simulink model "eVTOL_PX4_2023b"  (R2024b)
settings: Solver=ode4  StartTime=0  StopTime=inf  FixedStep=0.01  RelTol=1e-3
values from neighbouring files (symbols this model uses):
  aDl =     [initdata.mat]
  aDr =     [initdata.mat]
  aDyn =     [initdata.mat]
  Airport = init_airport('PHNL')    [initdata_HIL_eVTOL.m]
  aLat =     [initdata.mat]
  aLon =     [initdata.mat]
  D = Prop.D    [EOM_dt_MC.m]    (also in EOM_get_alf_dt_de_prop_evtol.m = CD * QS)
  dt0 = X(2)    [EOM_get_alf_dt_de_prop_evtol.m]    (also in initdata.mat = 0.258252593971; initdata_HIL_eVTOL.m = EOM_dt_MC)
  EAS0 = TAS0 / EAS2TAS    [initdata_HIL_eVTOL.m]
  FCS = init_FCS    [initdata_HIL_eVTOL.m]
  General = init_layoutdata    [EOM_dt_MC.m]    (also in build_optimized_CA.m; initdata.mat = ; initdata_HIL_eVTOL.m)
  h0 = Con(1)    [EOM_get_alf_dt_de_prop_evtol.m]    (also in initdata.mat = 450; initdata_HIL_eVTOL.m = 50)
  mass = Con(3)    [EOM_get_alf_dt_de_prop_evtol.m]    (also in initdata.mat = 2255.54; initdata_HIL_eVTOL.m = 7)
  Motor = init_motor_evtol    [EOM_dt_MC.m]    (also in initdata.mat = []; initdata_HIL_eVTOL.m)
  Prop = init_propeller_evtol_new    [EOM_dt_MC.m]    (also in initdata_HIL_eVTOL.m)
  R2D = 180/pi    (= 57.2957795131)    [EOM_get_alf_dt_de_prop_evtol.m]    (also in init_FCS.m; init_aerodata_evtol.m; init_airport.m; initdata.mat)
  SAMPLE_TIME = 0.01    [initdata_HIL_eVTOL.m]
  theta0 = -0.0510981441662    [initdata.mat]
undefined symbols (not defined in the file or in its folder): A1, aDa, aDe, aero, asbhl20env, B1, C1, de0, Earth, Environment, INIT_Data, InitData, Kd, Kp, magnitude, Newton, pProp, Raphson, Tc, WGS84
libraries: simulink_extras x63, vrlib x48, sharedtransform x28, simulink x22, slpidlib x20, sharedutil x20, matrix_library x18, aerolibwindfilters x12, aerolibobsolete x8, aerolibasang x8, aerolibatmos2 x6, aerolibfltsims x6
(part 16 of 17)

== system eVTOL_PX4_2023b/Subsystem2/airframe/force moment/aero F&M in body axis/Aerodynamic Coefficients/Body Rate Damping ==
  Incid : Inport
  pqrn : Inport  Port=2
  alphaDot_n : Inport  Port=3
  1-D Lookup Table : Lookup_n-D  NumberOfTableDimensions=1  BreakpointsForDimension1=aDyn.alpha  BreakpointsForDimension2=aDyn.flap  Table=aDyn.CYp  InternalRulePriority=Speed  RndMeth=Simplest
  1-D Lookup Table1 : Lookup_n-D  NumberOfTableDimensions=1  BreakpointsForDimension1=aDyn.alpha  BreakpointsForDimension2=aDyn.flap  Table=aDyn.Clp  InternalRulePriority=Speed  RndMeth=Simplest
  1-D Lookup Table2 : Lookup_n-D  NumberOfTableDimensions=1  BreakpointsForDimension1=aDyn.alpha  BreakpointsForDimension2=aDyn.flap  Table=aDyn.Cnp  InternalRulePriority=Speed  RndMeth=Simplest
  1-D Lookup Table3 : Lookup_n-D  NumberOfTableDimensions=1  BreakpointsForDimension1=aDyn.alpha  BreakpointsForDimension2=aDyn.flap  Table=aDyn.CYr  InternalRulePriority=Speed  RndMeth=Simplest
  1-D Lookup Table4 : Lookup_n-D  NumberOfTableDimensions=1  BreakpointsForDimension1=aDyn.alpha  BreakpointsForDimension2=aDyn.flap  Table=aDyn.Clr  InternalRulePriority=Speed  RndMeth=Simplest
  1-D Lookup Table5 : Lookup_n-D  NumberOfTableDimensions=1  BreakpointsForDimension1=aDyn.alpha  BreakpointsForDimension2=aDyn.flap  Table=aDyn.Cnr  InternalRulePriority=Speed  RndMeth=Simplest
  1-D Lookup Table6 : Lookup_n-D  NumberOfTableDimensions=1  BreakpointsForDimension1=aDyn.alpha  BreakpointsForDimension2=aDyn.flap  Table=aDyn.CLq  InternalRulePriority=Speed  RndMeth=Simplest
  1-D Lookup Table7 : Lookup_n-D  NumberOfTableDimensions=1  BreakpointsForDimension1=aDyn.alpha  BreakpointsForDimension2=aDyn.flap  Table=aDyn.Cmq  InternalRulePriority=Speed  RndMeth=Simplest
  1-D Lookup Table8 : Lookup_n-D  NumberOfTableDimensions=1  BreakpointsForDimension1=aDyn.alpha  BreakpointsForDimension2=aDyn.flap  Table=aDyn.CLAlphaDot  InternalRulePriority=Speed  RndMeth=Simplest
  1-D Lookup Table9 : Lookup_n-D  NumberOfTableDimensions=1  BreakpointsForDimension1=aDyn.alpha  BreakpointsForDimension2=aDyn.flap  Table=aDyn.CmAlphaDot  InternalRulePriority=Speed  RndMeth=Simplest
  Add : Sum  Inputs=++++
  Constant{,6..7,13} (4 alike) : Constant  Value=0
  Demux : Demux  Outputs=3
  Demux1 : Demux  Outputs=2
  Mux{1..4} (4 alike) : Mux  Inputs=6
  Product{4..7} (4 alike) : Product  InputSameDT=on  SaturateOnIntegerOverflow=on  OutDataTypeStr=Inherit: Same as first input
  Terminator : Terminator
  cl : Outport  InitialOutput=0  VectorParamsAs1DForOutWhenUnconnected=off
  wires:
  Add/1 -> cl/1
  1-D Lookup Table/1 -> Mux1/3  "CYp"
  1-D Lookup Table2/1 -> Mux1/6  "Cnp"
  Mux1/1 -> Product4/1
  1-D Lookup Table1/1 -> Mux1/4  "Clp"
  pqrn/1 -> Demux/1
  Demux/1 -> [p]
  Demux/2 -> [q]
  Demux/3 -> [r]
  Constant/1 -> Mux1/1, Mux1/2, Mux1/5
  1-D Lookup Table7/1 -> Mux2/5  "Cmq"
  1-D Lookup Table6/1 -> Mux2/1  "CLq"
  Mux2/1 -> Product5/1
  1-D Lookup Table3/1 -> Mux3/3  "CYr"
  Mux3/1 -> Product6/1
  1-D Lookup Table4/1 -> Mux3/4  "Clr"
  1-D Lookup Table5/1 -> Mux3/6  "Cnr"
  Constant7/1 -> Mux3/2, Mux3/5, Mux3/1
  Constant13/1 -> Mux4/6, Mux4/4, Mux4/3, Mux4/2
  1-D Lookup Table9/1 -> Mux4/5  "CmAlphaDot"
  1-D Lookup Table8/1 -> Mux4/1  "CLAlphaDot"
  Constant6/1 -> Mux2/4, Mux2/6, Mux2/3, Mux2/2
  [p] -> Product4/2
  [q] -> Product5/2
  [r] -> Product6/2
  Mux4/1 -> Product7/1
  alphaDot_n/1 -> Product7/2
  Product4/1 -> Add/1
  Product7/1 -> Add/4
  Demux1/2 -> Terminator/1  "beta"
  Demux1/1 -> [alpha]  "alpha"
  Incid/1 -> Demux1/1
  Product5/1 -> Add/3
  [alpha] -> 1-D Lookup Table3/1, 1-D Lookup Table4/1, 1-D Lookup Table9/1, 1-D Lookup Table8/1, 1-D Lookup Table7/1, 1-D Lookup Table6/1, 1-D Lookup Table5/1, 1-D Lookup Table2/1, 1-D Lookup Table1/1, 1-D Lookup Table/1
  Product6/1 -> Add/2

== system eVTOL_PX4_2023b/Subsystem2/airframe/force moment/aero F&M in body axis/Aerodynamic Coefficients/CLCDCY-CXCYCZ ==
  Incid : Inport
  Cl_LDY : Inport  Port=2
  Cl_xA : Fcn  Expr=-u[4]*cos(u[2])*cos(u[1])+u[3]*sin(u[1])
  Cl_yA : Fcn  Expr=-u[4]*sin(u[2])+u[5]
  Cl_zA : Fcn  Expr=-u[4]*cos(u[2])*sin(u[1])-u[3]*cos(u[1])
  Mux : Mux  Inputs=3
  Mux1 : Mux  Inputs=2
  Cl_XYZ : Outport  VectorParamsAs1DForOutWhenUnconnected=off
  wires:
  Mux/1 -> Cl_XYZ/1
  Cl_LDY/1 -> Mux1/2
  Incid/1 -> Mux1/1
  Cl_zA/1 -> Mux/3
  Cl_yA/1 -> Mux/2
  Cl_xA/1 -> Mux/1
  Mux1/1 -> Cl_zA/1, Cl_yA/1, Cl_xA/1

== system eVTOL_PX4_2023b/UAV/airframe/force moment/aero F&M in body axis/Aerodynamic Coefficients/Actuator Increments ==
  Actuators : Inport
  Aileron : Subsystem
  Bus Selector1 : BusSelector  OutputSignals=de,da,dr
  Elevator : Subsystem
  Ruder : Subsystem
  Sum : Sum  Inputs=+++
  da : Constant  Value=-1.25/57.3
  dr : Constant  Value=-6.3/57.3
  cl : Outport  InitialOutput=0  VectorParamsAs1DForOutWhenUnconnected=off
  wires:
  Actuators/1 -> Bus Selector1/1
  Bus Selector1/2 -> Aileron/1(da)  "<da>"
  Sum/1 -> cl/1
  Ruder/1(drCoeff) -> Sum/3
  Elevator/1(deCoeff) -> Sum/1
  Aileron/1(drCoeff) -> Sum/2
  Bus Selector1/1 -> Elevator/1(de)  "<de>"
  Bus Selector1/3 -> Ruder/1(dr)  "<dr>"

== system eVTOL_PX4_2023b/UAV/airframe/force moment/aero F&M in body axis/Aerodynamic Coefficients/Basic Coefficients ==
  Incid : Inport
  Constant : Constant  Value=aero.CL0
  Constant1 : Constant  Value=0
  Constant2 : Constant  Value=aero.CD0
  Constant3 : Constant  Value=aero.Cm0
  Constant4 : Constant  Value=0
  Demux : Demux  Outputs=2
  Gain : Gain  Gain=aero.CLAlpha
  Gain1 : Gain  Gain=aero.k
  Gain2 : Gain  Gain=aero.CmAlpha
  Gain3 : Gain  Gain=aero.CYBeta
  Gain4 : Gain  Gain=aero.ClBeta
  Gain5 : Gain  Gain=aero.CnBeta
  Mux1 : Mux  Inputs=6
  Mux2 : Mux  Inputs=6
  Product : Product
  Saturation : Saturate
  Saturation1 : Saturate  LowerLimit=-0.3
  Saturation2 : Saturate  UpperLimit=aero.CLMax  LowerLimit=-aero.CLMax
  Sum1 : Sum  Inputs=++|  InputSameDT=on  SaturateOnIntegerOverflow=on  OutDataTypeStr=Inherit: Same as first input
  Sum2 : Sum  Inputs=++|  InputSameDT=on  SaturateOnIntegerOverflow=on  OutDataTypeStr=Inherit: Same as first input
  Sum3 : Sum  Inputs=++|  InputSameDT=on  SaturateOnIntegerOverflow=on  OutDataTypeStr=Inherit: Same as first input
  Sum5 : Sum  Inputs=|++  InputSameDT=on  SaturateOnIntegerOverflow=on  OutDataTypeStr=Inherit: Same as first input
  cl : Outport  InitialOutput=0  VectorParamsAs1DForOutWhenUnconnected=off
  wires:
  Mux1/1 -> Sum5/1
  Demux/1 -> Saturation1/1  "alpha"
  Demux/2 -> Saturation/1  "beta"
  Sum2/1 -> Mux1/2
  Sum3/1 -> Mux1/5
  Sum1/1 -> Product/2, Product/1, Saturation2/1
  Constant1/1 -> Mux1/6, Mux1/4, Mux1/3
  Constant4/1 -> Mux2/5, Mux2/2, Mux2/1
  Gain3/1 -> Mux2/3
  Gain4/1 -> Mux2/4
  Gain5/1 -> Mux2/6
  Sum5/1 -> cl/1
  Mux2/1 -> Sum5/2
  Incid/1 -> Demux/1
  Saturation1/1 -> Gain2/1, Gain/1
  Saturation/1 -> Gain3/1, Gain5/1, Gain4/1
  Gain/1 -> Sum1/2
  Constant/1 -> Sum1/1
  Constant2/1 -> Sum2/1
  Product/1 -> Gain1/1
  Gain1/1 -> Sum2/2
  Constant3/1 -> Sum3/1
  Gain2/1 -> Sum3/2
  Saturation2/1 -> Mux1/1

== system eVTOL_PX4_2023b/UAV/airframe/force moment/aero F&M in body axis/Aerodynamic Coefficients/Body Rate Damping ==
  pqrn : Inport
  alphaDot_n : Inport  Port=2
  Demux : Demux  Outputs=3
  Product{,1..3} (4 alike) : Product  InputSameDT=on  SaturateOnIntegerOverflow=on  OutDataTypeStr=Inherit: Same as first input
  Sum1 : Sum  Inputs=++++  InputSameDT=on  SaturateOnIntegerOverflow=on  OutDataTypeStr=Inherit: Same as first input
  alphaDot : Subsystem
  p : Subsystem
  q : Subsystem
  r : Subsystem
  cl : Outport  InitialOutput=0  VectorParamsAs1DForOutWhenUnconnected=off
  wires:
  p/1(delCoeff) -> Product/1
  q/1(delCoeff) -> Product1/1
  Sum1/1 -> cl/1
  Product2/1 -> Sum1/3
  Product/1 -> Sum1/1
  r/1(delCoeff) -> Product2/1
  pqrn/1 -> Demux/1
  Demux/1 -> Product/2
  Demux/2 -> Product1/2
  Demux/3 -> Product2/2
  Product1/1 -> Sum1/2
  alphaDot/1(delCoeff) -> Product3/1
  alphaDot_n/1 -> Product3/2
  Product3/1 -> Sum1/4

== system eVTOL_PX4_2023b/UAV/airframe/force moment/aero F&M in body axis/Aerodynamic Coefficients/body axis forces ?????????? ==
  Incid : Inport
  Cl_LDY : Inport  Port=2
  Cl_xA : Fcn  Expr=-u[4]*cos(u[2])*cos(u[1])+u[3]*sin(u[1])
  Cl_yA : Fcn  Expr=-u[4]*sin(u[2])+u[5]
  Cl_zA : Fcn  Expr=-u[4]*cos(u[2])*sin(u[1])-u[3]*cos(u[1])
  Mux : Mux  Inputs=3
  Mux1 : Mux  Inputs=2
  Cl_XYZ : Outport  VectorParamsAs1DForOutWhenUnconnected=off
  wires:
  Mux/1 -> Cl_XYZ/1
  Cl_LDY/1 -> Mux1/2
  Incid/1 -> Mux1/1
  Cl_zA/1 -> Mux/3
  Cl_yA/1 -> Mux/2
  Cl_xA/1 -> Mux/1
  Mux1/1 -> Cl_zA/1, Cl_yA/1, Cl_xA/1

== system eVTOL_PX4_2023b/Subsystem1/Environment/Wind Models/Dryden Wind Turbulence Model (Continuous (+q -r))/Select angular rates/Interpolate rates/wind to body transformation ==
  DCM : Inport
  Wind direction : Inport  Port=2
  pg_l,qg_l,rg_l : Inport  Port=3
  Demux : Demux  Outputs=3
      settings: DisplayOption=none
  Product : Product  Multiplication=Matrix(*)  SaturateOnIntegerOverflow=on  OutDataTypeStr=Inherit: Same as first input
  Reshape : Reshape  OutputDimensionality=Customize  OutputDimensions=[3,1]
  Reshape1 : Reshape
  Vector Concatenate : Concatenate  NumInputs=3
  convert to earth coords : Subsystem
  pg,qg,rg : Outport  VectorParamsAs1DForOutWhenUnconnected=off
  wires:
  Reshape1/1 -> pg,qg,rg/1
  Reshape/1 -> Product/2
  DCM/1 -> Product/1
  Wind direction/1 -> convert to earth coords/1(Wind direction)
  convert to earth coords/1(pg) -> Vector Concatenate/1
  convert to earth coords/2(qg) -> Vector Concatenate/2
  Vector Concatenate/1 -> Reshape/1
  Demux/1 -> convert to earth coords/2(pg_l)
  Demux/2 -> convert to earth coords/3(qg_l)
  Demux/3 -> Vector Concatenate/3
  Product/1 -> Reshape1/1
  pg_l,qg_l,rg_l/1 -> Demux/1

== system eVTOL_PX4_2023b/Subsystem1/Environment/Wind Models/Dryden Wind Turbulence Model (Continuous (+q -r))/Select angular rates/Low altitude rates/wind to body transformation ==
  DCM : Inport
  Wind direction : Inport  Port=2
  pg_l,qg_l,rg_l : Inport  Port=3
  Demux : Demux  Outputs=3
      settings: DisplayOption=none
  Product : Product  Multiplication=Matrix(*)  SaturateOnIntegerOverflow=on  OutDataTypeStr=Inherit: Same as first input
  Reshape : Reshape  OutputDimensionality=Column vector (2-D)
  Reshape1 : Reshape
  Vector Concatenate : Concatenate  NumInputs=3
  convert to earth coords : Subsystem
  pg,qg,rg : Outport  VectorParamsAs1DForOutWhenUnconnected=off
  wires:
  pg_l,qg_l,rg_l/1 -> Demux/1
  Product/1 -> Reshape1/1
  Demux/3 -> Vector Concatenate/3
  Demux/2 -> convert to earth coords/3(qg_l)
  Demux/1 -> convert to earth coords/2(pg_l)
  Vector Concatenate/1 -> Reshape/1
  convert to earth coords/2(qg) -> Vector Concatenate/2
  convert to earth coords/1(pg) -> Vector Concatenate/1
  Wind direction/1 -> convert to earth coords/1(Wind direction)
  DCM/1 -> Product/1
  Reshape/1 -> Product/2
  Reshape1/1 -> pg,qg,rg/1

== system eVTOL_PX4_2023b/Subsystem1/Environment/Wind Models/Dryden Wind Turbulence Model (Continuous (+q -r))/Select velocities/Interpolate velocities/wind to body transformation ==
  DCM : Inport
  Wind direction : Inport  Port=2
  ug_l,vg_l,wg_l : Inport  Port=3
  Demux : Demux  Outputs=3
      settings: DisplayOption=none
  Product : Product  Multiplication=Matrix(*)  SaturateOnIntegerOverflow=on  OutDataTypeStr=Inherit: Same as first input
  Reshape : Reshape  OutputDimensionality=Customize  OutputDimensions=[3,1]
  Reshape1 : Reshape
  Vector Concatenate : Concatenate  NumInputs=3
  convert to earth coords : Subsystem
  ug,vg,wg : Outport  VectorParamsAs1DForOutWhenUnconnected=off
  wires:
  Reshape1/1 -> ug,vg,wg/1
  Reshape/1 -> Product/2
  ug_l,vg_l,wg_l/1 -> Demux/1
  Product/1 -> Reshape1/1
  Demux/3 -> Vector Concatenate/3
  Demux/2 -> convert to earth coords/3(vg_l)
  Demux/1 -> convert to earth coords/2(ug_l)
  Vector Concatenate/1 -> Reshape/1
  convert to earth coords/2(vg) -> Vector Concatenate/2
  convert to earth coords/1(ug) -> Vector Concatenate/1
  Wind direction/1 -> convert to earth coords/1(Wind direction)
  DCM/1 -> Product/1

== system eVTOL_PX4_2023b/Subsystem1/Environment/Wind Models/Dryden Wind Turbulence Model (Continuous (+q -r))/Select velocities/Low altitude velocities/wind to body transformation ==
  DCM : Inport
  Wind direction : Inport  Port=2
  ug_l,vg_l,wg_l : Inport  Port=3
  Demux : Demux  Outputs=3
      settings: DisplayOption=none
  Product : Product  Multiplication=Matrix(*)  SaturateOnIntegerOverflow=on  OutDataTypeStr=Inherit: Same as first input
  Reshape : Reshape  OutputDimensionality=Column vector (2-D)
  Reshape1 : Reshape
  Vector Concatenate : Concatenate  NumInputs=3
  convert to earth coords : Subsystem
  ug,vg,wg : Outport  VectorParamsAs1DForOutWhenUnconnected=off
  wires:
  DCM/1 -> Product/1
  Wind direction/1 -> convert to earth coords/1(Wind direction)
  convert to earth coords/1(ug) -> Vector Concatenate/1
  convert to earth coords/2(vg) -> Vector Concatenate/2
  Vector Concatenate/1 -> Reshape/1
  Demux/1 -> convert to earth coords/2(ug_l)
  Demux/2 -> convert to earth coords/3(vg_l)
  Demux/3 -> Vector Concatenate/3
  Product/1 -> Reshape1/1
  ug_l,vg_l,wg_l/1 -> Demux/1
  Reshape/1 -> Product/2
  Reshape1/1 -> ug,vg,wg/1

== system eVTOL_PX4_2023b/Subsystem1/Environment/Wind Models/Dryden Wind Turbulence Model (Continuous (+q -r))/Turbulence scale lengths/Medium//High altitude scale length/Length Conversion ==
  in : Inport  Unit=m
  Unit Conversion : UnitConversion
  out : Outport  VectorParamsAs1DForOutWhenUnconnected=off
  wires:
  in/1 -> Unit Conversion/1
  Unit Conversion/1 -> out/1

== system eVTOL_PX4_2023b/Subsystem1/Environment1/Wind Models/Dryden Wind Turbulence Model (Continuous (+q -r))/Select angular rates/Interpolate rates/wind to body transformation ==
  DCM : Inport
  Wind direction : Inport  Port=2
  pg_l,qg_l,rg_l : Inport  Port=3
  Demux : Demux  Outputs=3
      settings: DisplayOption=none
  Product : Product  Multiplication=Matrix(*)  SaturateOnIntegerOverflow=on  OutDataTypeStr=Inherit: Same as first input
  Reshape : Reshape  OutputDimensionality=Customize  OutputDimensions=[3,1]
  Reshape1 : Reshape
  Vector Concatenate : Concatenate  NumInputs=3
  convert to earth coords : Subsystem
  pg,qg,rg : Outport  VectorParamsAs1DForOutWhenUnconnected=off
  wires:
  Reshape1/1 -> pg,qg,rg/1
  Reshape/1 -> Product/2
  DCM/1 -> Product/1
  Wind direction/1 -> convert to earth coords/1(Wind direction)
  convert to earth coords/1(pg) -> Vector Concatenate/1
  convert to earth coords/2(qg) -> Vector Concatenate/2
  Vector Concatenate/1 -> Reshape/1
  Demux/1 -> convert to earth coords/2(pg_l)
  Demux/2 -> convert to earth coords/3(qg_l)
  Demux/3 -> Vector Concatenate/3
  Product/1 -> Reshape1/1
  pg_l,qg_l,rg_l/1 -> Demux/1

== system eVTOL_PX4_2023b/Subsystem1/Environment1/Wind Models/Dryden Wind Turbulence Model (Continuous (+q -r))/Select angular rates/Low altitude rates/wind to body transformation ==
  DCM : Inport
  Wind direction : Inport  Port=2
  pg_l,qg_l,rg_l : Inport  Port=3
  Demux : Demux  Outputs=3
      settings: DisplayOption=none
  Product : Product  Multiplication=Matrix(*)  SaturateOnIntegerOverflow=on  OutDataTypeStr=Inherit: Same as first input
  Reshape : Reshape  OutputDimensionality=Column vector (2-D)
  Reshape1 : Reshape
  Vector Concatenate : Concatenate  NumInputs=3
  convert to earth coords : Subsystem
  pg,qg,rg : Outport  VectorParamsAs1DForOutWhenUnconnected=off
  wires:
  pg_l,qg_l,rg_l/1 -> Demux/1
  Product/1 -> Reshape1/1
  Demux/3 -> Vector Concatenate/3
  Demux/2 -> convert to earth coords/3(qg_l)
  Demux/1 -> convert to earth coords/2(pg_l)
  Vector Concatenate/1 -> Reshape/1
  convert to earth coords/2(qg) -> Vector Concatenate/2
  convert to earth coords/1(pg) -> Vector Concatenate/1
  Wind direction/1 -> convert to earth coords/1(Wind direction)
  DCM/1 -> Product/1
  Reshape/1 -> Product/2
  Reshape1/1 -> pg,qg,rg/1

== system eVTOL_PX4_2023b/Subsystem1/Environment1/Wind Models/Dryden Wind Turbulence Model (Continuous (+q -r))/Select velocities/Interpolate velocities/wind to body transformation ==
  DCM : Inport
  Wind direction : Inport  Port=2
  ug_l,vg_l,wg_l : Inport  Port=3
  Demux : Demux  Outputs=3
      settings: DisplayOption=none
  Product : Product  Multiplication=Matrix(*)  SaturateOnIntegerOverflow=on  OutDataTypeStr=Inherit: Same as first input
  Reshape : Reshape  OutputDimensionality=Customize  OutputDimensions=[3,1]
  Reshape1 : Reshape
  Vector Concatenate : Concatenate  NumInputs=3
  convert to earth coords : Subsystem
  ug,vg,wg : Outport  VectorParamsAs1DForOutWhenUnconnected=off
  wires:
  Reshape1/1 -> ug,vg,wg/1
  Reshape/1 -> Product/2
  ug_l,vg_l,wg_l/1 -> Demux/1
  Product/1 -> Reshape1/1
  Demux/3 -> Vector Concatenate/3
  Demux/2 -> convert to earth coords/3(vg_l)
  Demux/1 -> convert to earth coords/2(ug_l)
  Vector Concatenate/1 -> Reshape/1
  convert to earth coords/2(vg) -> Vector Concatenate/2
  convert to earth coords/1(ug) -> Vector Concatenate/1
  Wind direction/1 -> convert to earth coords/1(Wind direction)
  DCM/1 -> Product/1

== system eVTOL_PX4_2023b/Subsystem1/Environment1/Wind Models/Dryden Wind Turbulence Model (Continuous (+q -r))/Select velocities/Low altitude velocities/wind to body transformation ==
  DCM : Inport
  Wind direction : Inport  Port=2
  ug_l,vg_l,wg_l : Inport  Port=3
  Demux : Demux  Outputs=3
      settings: DisplayOption=none
  Product : Product  Multiplication=Matrix(*)  SaturateOnIntegerOverflow=on  OutDataTypeStr=Inherit: Same as first input
  Reshape : Reshape  OutputDimensionality=Column vector (2-D)
  Reshape1 : Reshape
  Vector Concatenate : Concatenate  NumInputs=3
  convert to earth coords : Subsystem
  ug,vg,wg : Outport  VectorParamsAs1DForOutWhenUnconnected=off
  wires:
  DCM/1 -> Product/1
  Wind direction/1 -> convert to earth coords/1(Wind direction)
  convert to earth coords/1(ug) -> Vector Concatenate/1
  convert to earth coords/2(vg) -> Vector Concatenate/2
  Vector Concatenate/1 -> Reshape/1
  Demux/1 -> convert to earth coords/2(ug_l)
  Demux/2 -> convert to earth coords/3(vg_l)
  Demux/3 -> Vector Concatenate/3
  Product/1 -> Reshape1/1
  ug_l,vg_l,wg_l/1 -> Demux/1
  Reshape/1 -> Product/2
  Reshape1/1 -> ug,vg,wg/1

== system eVTOL_PX4_2023b/Subsystem1/Environment1/Wind Models/Dryden Wind Turbulence Model (Continuous (+q -r))/Turbulence scale lengths/Medium//High altitude scale length/Length Conversion ==
  in : Inport  Unit=m
  Unit Conversion : UnitConversion
  out : Outport  VectorParamsAs1DForOutWhenUnconnected=off
  wires:
  in/1 -> Unit Conversion/1
  Unit Conversion/1 -> out/1

== system eVTOL_PX4_2023b/Subsystem1/airframe/force moment/aero F&M in body axis/Aerodynamic Coefficients/Actuator Increments/Aileron ==
  alpha : Inport
  da : Inport  Port=2
  2-D Lookup Table3 : Lookup_n-D  NumberOfTableDimensions=1  BreakpointsForDimension1=aDa.alpha  BreakpointsForDimension2=aDe.alpha  BreakpointsForDimension3=aDe.flap  Table=aDa.CYDa  InternalRulePriority=Speed  RndMeth=Simplest
  2-D Lookup Table4 : Lookup_n-D  NumberOfTableDimensions=1  BreakpointsForDimension1=aDa.alpha  BreakpointsForDimension2=aDe.alpha  BreakpointsForDimension3=aDe.flap  Table=aDa.ClDa  InternalRulePriority=Speed  RndMeth=Simplest
  2-D Lookup Table5 : Lookup_n-D  NumberOfTableDimensions=1  BreakpointsForDimension1=aDa.alpha  BreakpointsForDimension2=aDe.alpha  BreakpointsForDimension3=aDe.flap  Table=aDa.CnDa  InternalRulePriority=Speed  RndMeth=Simplest
  Constant : Constant  Value=0
  Divide2 : Product  Inputs=**
  Divide3 : Product  Inputs=**
  Divide5 : Product  Inputs=**
  Mux1 : Mux  Inputs=6
  Saturation : Saturate  UpperLimit=12/57.3  LowerLimit=-4/57.3
  da_Coeff : Outport  VectorParamsAs1DForOutWhenUnconnected=off
  wires:
  alpha/1 -> Saturation/1
  Mux1/1 -> da_Coeff/1
  da/1 -> Divide5/1, Divide3/1, Divide2/1
  Divide2/1 -> Mux1/3
  Divide3/1 -> Mux1/4
  2-D Lookup Table3/1 -> Divide2/2
  Divide5/1 -> Mux1/6
  2-D Lookup Table5/1 -> Divide5/2
  2-D Lookup Table4/1 -> Divide3/2
  Constant/1 -> Mux1/5, Mux1/2, Mux1/1
  Saturation/1 -> 2-D Lookup Table5/1, 2-D Lookup Table4/1, 2-D Lookup Table3/1

== system eVTOL_PX4_2023b/Subsystem1/airframe/force moment/aero F&M in body axis/Aerodynamic Coefficients/Actuator Increments/V_left ==
  alpha : Inport
  dl : Inport  Port=2
  2-D Lookup Table : Lookup_n-D  NumberOfTableDimensions=1  BreakpointsForDimension1=aDl.alpha  BreakpointsForDimension2=aDl.alpha  BreakpointsForDimension3=aDe.flap  Table=aDl.CLDl  InternalRulePriority=Speed  RndMeth=Simplest
  2-D Lookup Table1 : Lookup_n-D  NumberOfTableDimensions=1  BreakpointsForDimension1=aDl.alpha  BreakpointsForDimension2=aDe.alpha  BreakpointsForDimension3=aDe.flap  Table=aDl.CmDl  InternalRulePriority=Speed  RndMeth=Simplest
  2-D Lookup Table2 : Lookup_n-D  NumberOfTableDimensions=1  BreakpointsForDimension1=aDl.alpha  BreakpointsForDimension2=aDe.alpha  BreakpointsForDimension3=aDe.flap  Table=aDl.CDDl  InternalRulePriority=Speed  RndMeth=Simplest
  2-D Lookup Table3 : Lookup_n-D  NumberOfTableDimensions=1  BreakpointsForDimension1=aDl.alpha  BreakpointsForDimension2=aDe.alpha  BreakpointsForDimension3=aDe.flap  Table=aDl.CYDl  InternalRulePriority=Speed  RndMeth=Simplest
  2-D Lookup Table4 : Lookup_n-D  NumberOfTableDimensions=1  BreakpointsForDimension1=aDl.alpha  BreakpointsForDimension2=aDe.alpha  BreakpointsForDimension3=aDe.flap  Table=aDl.ClDl  InternalRulePriority=Speed  RndMeth=Simplest
  2-D Lookup Table5 : Lookup_n-D  NumberOfTableDimensions=1  BreakpointsForDimension1=aDl.alpha  BreakpointsForDimension2=aDe.alpha  BreakpointsForDimension3=aDe.flap  Table=aDl.CnDl  InternalRulePriority=Speed  RndMeth=Simplest
  Divide{,1..5} (6 alike) : Product  Inputs=**
  Mux1 : Mux  Inputs=6
  Saturation : Saturate  UpperLimit=12/57.3  LowerLimit=-4/57.3
  dl_Coeff : Outport  VectorParamsAs1DForOutWhenUnconnected=off
  wires:
  2-D Lookup Table/1 -> Divide/2
  2-D Lookup Table2/1 -> Divide1/2
  2-D Lookup Table1/1 -> Divide4/2
  Mux1/1 -> dl_Coeff/1
  Divide4/1 -> Mux1/5
  Divide/1 -> Mux1/1
  Divide1/1 -> Mux1/2
  Divide2/1 -> Mux1/3
  2-D Lookup Table3/1 -> Divide2/2
  Divide3/1 -> Mux1/4
  2-D Lookup Table4/1 -> Divide3/2
  dl/1 -> Divide5/1, Divide4/1, Divide3/1, Divide2/1, Divide1/1, Divide/1
  alpha/1 -> Saturation/1
  2-D Lookup Table5/1 -> Divide5/2
  Divide5/1 -> Mux1/6
  Saturation/1 -> 2-D Lookup Table5/1, 2-D Lookup Table1/1, 2-D Lookup Table4/1, 2-D Lookup Table3/1, 2-D Lookup Table2/1, 2-D Lookup Table/1

== system eVTOL_PX4_2023b/Subsystem1/airframe/force moment/aero F&M in body axis/Aerodynamic Coefficients/Actuator Increments/V_right ==
  alpha : Inport
  dr : Inport  Port=2
  2-D Lookup Table : Lookup_n-D  NumberOfTableDimensions=1  BreakpointsForDimension1=aDr.alpha  BreakpointsForDimension2=aDl.alpha  BreakpointsForDimension3=aDe.flap  Table=aDr.CLDr  InternalRulePriority=Speed  RndMeth=Simplest
  2-D Lookup Table1 : Lookup_n-D  NumberOfTableDimensions=1  BreakpointsForDimension1=aDr.alpha  BreakpointsForDimension2=aDe.alpha  BreakpointsForDimension3=aDe.flap  Table=aDr.CmDr  InternalRulePriority=Speed  RndMeth=Simplest
  2-D Lookup Table2 : Lookup_n-D  NumberOfTableDimensions=1  BreakpointsForDimension1=aDr.alpha  BreakpointsForDimension2=aDe.alpha  BreakpointsForDimension3=aDe.flap  Table=aDr.CDDr  InternalRulePriority=Speed  RndMeth=Simplest
  2-D Lookup Table3 : Lookup_n-D  NumberOfTableDimensions=1  BreakpointsForDimension1=aDr.alpha  BreakpointsForDimension2=aDe.alpha  BreakpointsForDimension3=aDe.flap  Table=aDr.CYDr  InternalRulePriority=Speed  RndMeth=Simplest
  2-D Lookup Table4 : Lookup_n-D  NumberOfTableDimensions=1  BreakpointsForDimension1=aDr.alpha  BreakpointsForDimension2=aDe.alpha  BreakpointsForDimension3=aDe.flap  Table=aDr.ClDr  InternalRulePriority=Speed  RndMeth=Simplest
  2-D Lookup Table5 : Lookup_n-D  NumberOfTableDimensions=1  BreakpointsForDimension1=aDr.alpha  BreakpointsForDimension2=aDe.alpha  BreakpointsForDimension3=aDe.flap  Table=aDr.CnDr  InternalRulePriority=Speed  RndMeth=Simplest
  Divide{,1..5} (6 alike) : Product  Inputs=**
  Mux1 : Mux  Inputs=6
  Saturation : Saturate  UpperLimit=12/57.3  LowerLimit=-4/57.3
  dr_Coeff : Outport  VectorParamsAs1DForOutWhenUnconnected=off
  wires:
  dr/1 -> Divide5/1, Divide4/1, Divide3/1, Divide2/1, Divide1/1, Divide/1
  alpha/1 -> Saturation/1
  Divide/1 -> Mux1/1
  2-D Lookup Table5/1 -> Divide5/2
  Divide5/1 -> Mux1/6
  2-D Lookup Table1/1 -> Divide4/2
  Divide4/1 -> Mux1/5
  Divide2/1 -> Mux1/3
  2-D Lookup Table4/1 -> Divide3/2
  2-D Lookup Table/1 -> Divide/2
  2-D Lookup Table3/1 -> Divide2/2
  Mux1/1 -> dr_Coeff/1
  Divide3/1 -> Mux1/4
  2-D Lookup Table2/1 -> Divide1/2
  Divide1/1 -> Mux1/2
  Saturation/1 -> 2-D Lookup Table5/1, 2-D Lookup Table1/1, 2-D Lookup Table4/1, 2-D Lookup Table3/1, 2-D Lookup Table2/1, 2-D Lookup Table/1

== system eVTOL_PX4_2023b/Subsystem1/airframe1/force moment/aero F&M in body axis/Aerodynamic Coefficients/Actuator Increments/Aileron ==
  alpha : Inport
  da : Inport  Port=2
  2-D Lookup Table3 : Lookup_n-D  NumberOfTableDimensions=1  BreakpointsForDimension1=aDa.alpha  BreakpointsForDimension2=aDe.alpha  BreakpointsForDimension3=aDe.flap  Table=aDa.CYDa  InternalRulePriority=Speed  RndMeth=Simplest
  2-D Lookup Table4 : Lookup_n-D  NumberOfTableDimensions=1  BreakpointsForDimension1=aDa.alpha  BreakpointsForDimension2=aDe.alpha  BreakpointsForDimension3=aDe.flap  Table=aDa.ClDa  InternalRulePriority=Speed  RndMeth=Simplest
  2-D Lookup Table5 : Lookup_n-D  NumberOfTableDimensions=1  BreakpointsForDimension1=aDa.alpha  BreakpointsForDimension2=aDe.alpha  BreakpointsForDimension3=aDe.flap  Table=aDa.CnDa  InternalRulePriority=Speed  RndMeth=Simplest
  Constant : Constant  Value=0
  Divide2 : Product  Inputs=**
  Divide3 : Product  Inputs=**
  Divide5 : Product  Inputs=**
  Mux1 : Mux  Inputs=6
  da_Coeff : Outport  VectorParamsAs1DForOutWhenUnconnected=off
  wires:
  alpha/1 -> 2-D Lookup Table5/1, 2-D Lookup Table4/1, 2-D Lookup Table3/1
  Mux1/1 -> da_Coeff/1
  da/1 -> Divide5/1, Divide3/1, Divide2/1
  Divide2/1 -> Mux1/3
  Divide3/1 -> Mux1/4
  2-D Lookup Table3/1 -> Divide2/2
  Divide5/1 -> Mux1/6
  2-D Lookup Table5/1 -> Divide5/2
  2-D Lookup Table4/1 -> Divide3/2
  Constant/1 -> Mux1/5, Mux1/2, Mux1/1

== system eVTOL_PX4_2023b/Subsystem1/airframe1/force moment/aero F&M in body axis/Aerodynamic Coefficients/Actuator Increments/V_left ==
  alpha : Inport
  dl : Inport  Port=2
  2-D Lookup Table : Lookup_n-D  NumberOfTableDimensions=1  BreakpointsForDimension1=aDl.alpha  BreakpointsForDimension2=aDl.alpha  BreakpointsForDimension3=aDe.flap  Table=aDl.CLDl  InternalRulePriority=Speed  RndMeth=Simplest
  2-D Lookup Table1 : Lookup_n-D  NumberOfTableDimensions=1  BreakpointsForDimension1=aDl.alpha  BreakpointsForDimension2=aDe.alpha  BreakpointsForDimension3=aDe.flap  Table=aDl.CmDl  InternalRulePriority=Speed  RndMeth=Simplest
  2-D Lookup Table2 : Lookup_n-D  NumberOfTableDimensions=1  BreakpointsForDimension1=aDl.alpha  BreakpointsForDimension2=aDe.alpha  BreakpointsForDimension3=aDe.flap  Table=aDl.CDDl  InternalRulePriority=Speed  RndMeth=Simplest
  2-D Lookup Table3 : Lookup_n-D  NumberOfTableDimensions=1  BreakpointsForDimension1=aDl.alpha  BreakpointsForDimension2=aDe.alpha  BreakpointsForDimension3=aDe.flap  Table=aDl.CYDl  InternalRulePriority=Speed  RndMeth=Simplest
  2-D Lookup Table4 : Lookup_n-D  NumberOfTableDimensions=1  BreakpointsForDimension1=aDl.alpha  BreakpointsForDimension2=aDe.alpha  BreakpointsForDimension3=aDe.flap  Table=aDl.ClDl  InternalRulePriority=Speed  RndMeth=Simplest
  2-D Lookup Table5 : Lookup_n-D  NumberOfTableDimensions=1  BreakpointsForDimension1=aDl.alpha  BreakpointsForDimension2=aDe.alpha  BreakpointsForDimension3=aDe.flap  Table=aDl.CnDl  InternalRulePriority=Speed  RndMeth=Simplest
  Divide{,1..5} (6 alike) : Product  Inputs=**
  Mux1 : Mux  Inputs=6
  dl_Coeff : Outport  VectorParamsAs1DForOutWhenUnconnected=off
  wires:
  2-D Lookup Table/1 -> Divide/2
  2-D Lookup Table2/1 -> Divide1/2
  2-D Lookup Table1/1 -> Divide4/2
  Mux1/1 -> dl_Coeff/1
  Divide4/1 -> Mux1/5
  Divide/1 -> Mux1/1
  Divide1/1 -> Mux1/2
  Divide2/1 -> Mux1/3
  2-D Lookup Table3/1 -> Divide2/2
  Divide3/1 -> Mux1/4
  2-D Lookup Table4/1 -> Divide3/2
  dl/1 -> Divide5/1, Divide4/1, Divide3/1, Divide2/1, Divide1/1, Divide/1
  alpha/1 -> 2-D Lookup Table5/1, 2-D Lookup Table1/1, 2-D Lookup Table4/1, 2-D Lookup Table3/1, 2-D Lookup Table2/1, 2-D Lookup Table/1
  2-D Lookup Table5/1 -> Divide5/2
  Divide5/1 -> Mux1/6

== system eVTOL_PX4_2023b/Subsystem1/airframe1/force moment/aero F&M in body axis/Aerodynamic Coefficients/Actuator Increments/V_right ==
  alpha : Inport
  dr : Inport  Port=2
  2-D Lookup Table : Lookup_n-D  NumberOfTableDimensions=1  BreakpointsForDimension1=aDr.alpha  BreakpointsForDimension2=aDl.alpha  BreakpointsForDimension3=aDe.flap  Table=aDr.CLDr  InternalRulePriority=Speed  RndMeth=Simplest
  2-D Lookup Table1 : Lookup_n-D  NumberOfTableDimensions=1  BreakpointsForDimension1=aDr.alpha  BreakpointsForDimension2=aDe.alpha  BreakpointsForDimension3=aDe.flap  Table=aDr.CmDr  InternalRulePriority=Speed  RndMeth=Simplest
  2-D Lookup Table2 : Lookup_n-D  NumberOfTableDimensions=1  BreakpointsForDimension1=aDr.alpha  BreakpointsForDimension2=aDe.alpha  BreakpointsForDimension3=aDe.flap  Table=aDr.CDDr  InternalRulePriority=Speed  RndMeth=Simplest
  2-D Lookup Table3 : Lookup_n-D  NumberOfTableDimensions=1  BreakpointsForDimension1=aDr.alpha  BreakpointsForDimension2=aDe.alpha  BreakpointsForDimension3=aDe.flap  Table=aDr.CYDr  InternalRulePriority=Speed  RndMeth=Simplest
  2-D Lookup Table4 : Lookup_n-D  NumberOfTableDimensions=1  BreakpointsForDimension1=aDr.alpha  BreakpointsForDimension2=aDe.alpha  BreakpointsForDimension3=aDe.flap  Table=aDr.ClDr  InternalRulePriority=Speed  RndMeth=Simplest
  2-D Lookup Table5 : Lookup_n-D  NumberOfTableDimensions=1  BreakpointsForDimension1=aDr.alpha  BreakpointsForDimension2=aDe.alpha  BreakpointsForDimension3=aDe.flap  Table=aDr.CnDr  InternalRulePriority=Speed  RndMeth=Simplest
  Divide{,1..5} (6 alike) : Product  Inputs=**
  Mux1 : Mux  Inputs=6
  dr_Coeff : Outport  VectorParamsAs1DForOutWhenUnconnected=off
  wires:
  dr/1 -> Divide5/1, Divide4/1, Divide3/1, Divide2/1, Divide1/1, Divide/1
  alpha/1 -> 2-D Lookup Table5/1, 2-D Lookup Table1/1, 2-D Lookup Table4/1, 2-D Lookup Table3/1, 2-D Lookup Table2/1, 2-D Lookup Table/1
  Divide/1 -> Mux1/1
  2-D Lookup Table5/1 -> Divide5/2
  Divide5/1 -> Mux1/6
  2-D Lookup Table1/1 -> Divide4/2
  Divide4/1 -> Mux1/5
  Divide2/1 -> Mux1/3
  2-D Lookup Table4/1 -> Divide3/2
  2-D Lookup Table/1 -> Divide/2
  2-D Lookup Table3/1 -> Divide2/2
  Mux1/1 -> dr_Coeff/1
  Divide3/1 -> Mux1/4
  2-D Lookup Table2/1 -> Divide1/2
  Divide1/1 -> Mux1/2

== system eVTOL_PX4_2023b/Subsystem2/Environment/Wind Models/Dryden Wind Turbulence Model (Continuous (+q -r))/Select angular rates/Interpolate rates/wind to body transformation ==
  DCM : Inport
  Wind direction : Inport  Port=2
  pg_l,qg_l,rg_l : Inport  Port=3
  Demux : Demux  Outputs=3
      settings: DisplayOption=none
  Product : Product  Multiplication=Matrix(*)  SaturateOnIntegerOverflow=on  OutDataTypeStr=Inherit: Same as first input
  Reshape : Reshape  OutputDimensionality=Customize  OutputDimensions=[3,1]
  Reshape1 : Reshape
  Vector Concatenate : Concatenate  NumInputs=3
  convert to earth coords : Subsystem
  pg,qg,rg : Outport  VectorParamsAs1DForOutWhenUnconnected=off
  wires:
  Reshape1/1 -> pg,qg,rg/1
  Reshape/1 -> Product/2
  DCM/1 -> Product/1
  Wind direction/1 -> convert to earth coords/1(Wind direction)
  convert to earth coords/1(pg) -> Vector Concatenate/1
  convert to earth coords/2(qg) -> Vector Concatenate/2
  Vector Concatenate/1 -> Reshape/1
  Demux/1 -> convert to earth coords/2(pg_l)
  Demux/2 -> convert to earth coords/3(qg_l)
  Demux/3 -> Vector Concatenate/3
  Product/1 -> Reshape1/1
  pg_l,qg_l,rg_l/1 -> Demux/1

== system eVTOL_PX4_2023b/Subsystem2/Environment/Wind Models/Dryden Wind Turbulence Model (Continuous (+q -r))/Select angular rates/Low altitude rates/wind to body transformation ==
  DCM : Inport
  Wind direction : Inport  Port=2
  pg_l,qg_l,rg_l : Inport  Port=3
  Demux : Demux  Outputs=3
      settings: DisplayOption=none
  Product : Product  Multiplication=Matrix(*)  SaturateOnIntegerOverflow=on  OutDataTypeStr=Inherit: Same as first input
  Reshape : Reshape  OutputDimensionality=Column vector (2-D)
  Reshape1 : Reshape
  Vector Concatenate : Concatenate  NumInputs=3
  convert to earth coords : Subsystem
  pg,qg,rg : Outport  VectorParamsAs1DForOutWhenUnconnected=off
  wires:
  pg_l,qg_l,rg_l/1 -> Demux/1
  Product/1 -> Reshape1/1
  Demux/3 -> Vector Concatenate/3
  Demux/2 -> convert to earth coords/3(qg_l)
  Demux/1 -> convert to earth coords/2(pg_l)
  Vector Concatenate/1 -> Reshape/1
  convert to earth coords/2(qg) -> Vector Concatenate/2
  convert to earth coords/1(pg) -> Vector Concatenate/1
  Wind direction/1 -> convert to earth coords/1(Wind direction)
  DCM/1 -> Product/1
  Reshape/1 -> Product/2
  Reshape1/1 -> pg,qg,rg/1

== system eVTOL_PX4_2023b/Subsystem2/Environment/Wind Models/Dryden Wind Turbulence Model (Continuous (+q -r))/Select velocities/Interpolate velocities/wind to body transformation ==
  DCM : Inport
  Wind direction : Inport  Port=2
  ug_l,vg_l,wg_l : Inport  Port=3
  Demux : Demux  Outputs=3
      settings: DisplayOption=none
  Product : Product  Multiplication=Matrix(*)  SaturateOnIntegerOverflow=on  OutDataTypeStr=Inherit: Same as first input
  Reshape : Reshape  OutputDimensionality=Customize  OutputDimensions=[3,1]
  Reshape1 : Reshape
  Vector Concatenate : Concatenate  NumInputs=3
  convert to earth coords : Subsystem
  ug,vg,wg : Outport  VectorParamsAs1DForOutWhenUnconnected=off
  wires:
  Reshape1/1 -> ug,vg,wg/1
  Reshape/1 -> Product/2
  ug_l,vg_l,wg_l/1 -> Demux/1
  Product/1 -> Reshape1/1
  Demux/3 -> Vector Concatenate/3
  Demux/2 -> convert to earth coords/3(vg_l)
  Demux/1 -> convert to earth coords/2(ug_l)
  Vector Concatenate/1 -> Reshape/1
  convert to earth coords/2(vg) -> Vector Concatenate/2
  convert to earth coords/1(ug) -> Vector Concatenate/1
  Wind direction/1 -> convert to earth coords/1(Wind direction)
  DCM/1 -> Product/1

== system eVTOL_PX4_2023b/Subsystem2/Environment/Wind Models/Dryden Wind Turbulence Model (Continuous (+q -r))/Select velocities/Low altitude velocities/wind to body transformation ==
  DCM : Inport
  Wind direction : Inport  Port=2
  ug_l,vg_l,wg_l : Inport  Port=3
  Demux : Demux  Outputs=3
      settings: DisplayOption=none
  Product : Product  Multiplication=Matrix(*)  SaturateOnIntegerOverflow=on  OutDataTypeStr=Inherit: Same as first input
  Reshape : Reshape  OutputDimensionality=Column vector (2-D)
  Reshape1 : Reshape
  Vector Concatenate : Concatenate  NumInputs=3
  convert to earth coords : Subsystem
  ug,vg,wg : Outport  VectorParamsAs1DForOutWhenUnconnected=off
  wires:
  DCM/1 -> Product/1
  Wind direction/1 -> convert to earth coords/1(Wind direction)
  convert to earth coords/1(ug) -> Vector Concatenate/1
  convert to earth coords/2(vg) -> Vector Concatenate/2
  Vector Concatenate/1 -> Reshape/1
  Demux/1 -> convert to earth coords/2(ug_l)
  Demux/2 -> convert to earth coords/3(vg_l)
  Demux/3 -> Vector Concatenate/3
  Product/1 -> Reshape1/1
  ug_l,vg_l,wg_l/1 -> Demux/1
  Reshape/1 -> Product/2
  Reshape1/1 -> ug,vg,wg/1

== system eVTOL_PX4_2023b/Subsystem2/Environment/Wind Models/Dryden Wind Turbulence Model (Continuous (+q -r))/Turbulence scale lengths/Medium//High altitude scale length/Length Conversion ==
  in : Inport  Unit=m
  Unit Conversion : UnitConversion
  out : Outport  VectorParamsAs1DForOutWhenUnconnected=off
  wires:
  in/1 -> Unit Conversion/1
  Unit Conversion/1 -> out/1

== system eVTOL_PX4_2023b/Subsystem2/airframe/force moment/aero F&M in body axis/Aerodynamic Coefficients/Actuator Increments/Aileron ==
  alpha : Inport
  da : Inport  Port=2
  2-D Lookup Table3 : Lookup_n-D  NumberOfTableDimensions=1  BreakpointsForDimension1=aDa.alpha  BreakpointsForDimension2=aDe.alpha  BreakpointsForDimension3=aDe.flap  Table=aDa.CYDa  InternalRulePriority=Speed  RndMeth=Simplest
  2-D Lookup Table4 : Lookup_n-D  NumberOfTableDimensions=1  BreakpointsForDimension1=aDa.alpha  BreakpointsForDimension2=aDe.alpha  BreakpointsForDimension3=aDe.flap  Table=aDa.ClDa  InternalRulePriority=Speed  RndMeth=Simplest
  2-D Lookup Table5 : Lookup_n-D  NumberOfTableDimensions=1  BreakpointsForDimension1=aDa.alpha  BreakpointsForDimension2=aDe.alpha  BreakpointsForDimension3=aDe.flap  Table=aDa.CnDa  InternalRulePriority=Speed  RndMeth=Simplest
  Constant : Constant  Value=0
  Divide2 : Product  Inputs=**
  Divide3 : Product  Inputs=**
  Divide5 : Product  Inputs=**
  Mux1 : Mux  Inputs=6
  da_Coeff : Outport  VectorParamsAs1DForOutWhenUnconnected=off
  wires:
  alpha/1 -> 2-D Lookup Table5/1, 2-D Lookup Table4/1, 2-D Lookup Table3/1
  Mux1/1 -> da_Coeff/1
  da/1 -> Divide5/1, Divide3/1, Divide2/1
  Divide2/1 -> Mux1/3
  Divide3/1 -> Mux1/4
  2-D Lookup Table3/1 -> Divide2/2
  Divide5/1 -> Mux1/6
  2-D Lookup Table5/1 -> Divide5/2
  2-D Lookup Table4/1 -> Divide3/2
  Constant/1 -> Mux1/5, Mux1/2, Mux1/1

== system eVTOL_PX4_2023b/Subsystem2/airframe/force moment/aero F&M in body axis/Aerodynamic Coefficients/Actuator Increments/V_left ==
  alpha : Inport
  dl : Inport  Port=2
  2-D Lookup Table : Lookup_n-D  NumberOfTableDimensions=1  BreakpointsForDimension1=aDl.alpha  BreakpointsForDimension2=aDl.alpha  BreakpointsForDimension3=aDe.flap  Table=aDl.CLDl  InternalRulePriority=Speed  RndMeth=Simplest
  2-D Lookup Table1 : Lookup_n-D  NumberOfTableDimensions=1  BreakpointsForDimension1=aDl.alpha  BreakpointsForDimension2=aDe.alpha  BreakpointsForDimension3=aDe.flap  Table=aDl.CmDl  InternalRulePriority=Speed  RndMeth=Simplest
  2-D Lookup Table2 : Lookup_n-D  NumberOfTableDimensions=1  BreakpointsForDimension1=aDl.alpha  BreakpointsForDimension2=aDe.alpha  BreakpointsForDimension3=aDe.flap  Table=aDl.CDDl  InternalRulePriority=Speed  RndMeth=Simplest
  2-D Lookup Table3 : Lookup_n-D  NumberOfTableDimensions=1  BreakpointsForDimension1=aDl.alpha  BreakpointsForDimension2=aDe.alpha  BreakpointsForDimension3=aDe.flap  Table=aDl.CYDl  InternalRulePriority=Speed  RndMeth=Simplest
  2-D Lookup Table4 : Lookup_n-D  NumberOfTableDimensions=1  BreakpointsForDimension1=aDl.alpha  BreakpointsForDimension2=aDe.alpha  BreakpointsForDimension3=aDe.flap  Table=aDl.ClDl  InternalRulePriority=Speed  RndMeth=Simplest
  2-D Lookup Table5 : Lookup_n-D  NumberOfTableDimensions=1  BreakpointsForDimension1=aDl.alpha  BreakpointsForDimension2=aDe.alpha  BreakpointsForDimension3=aDe.flap  Table=aDl.CnDl  InternalRulePriority=Speed  RndMeth=Simplest
  Divide{,1..5} (6 alike) : Product  Inputs=**
  Mux1 : Mux  Inputs=6
  dl_Coeff : Outport  VectorParamsAs1DForOutWhenUnconnected=off
  wires:
  2-D Lookup Table/1 -> Divide/2
  2-D Lookup Table2/1 -> Divide1/2
  2-D Lookup Table1/1 -> Divide4/2
  Mux1/1 -> dl_Coeff/1
  Divide4/1 -> Mux1/5
  Divide/1 -> Mux1/1
  Divide1/1 -> Mux1/2
  Divide2/1 -> Mux1/3
  2-D Lookup Table3/1 -> Divide2/2
  Divide3/1 -> Mux1/4
  2-D Lookup Table4/1 -> Divide3/2
  dl/1 -> Divide5/1, Divide4/1, Divide3/1, Divide2/1, Divide1/1, Divide/1
  alpha/1 -> 2-D Lookup Table5/1, 2-D Lookup Table1/1, 2-D Lookup Table4/1, 2-D Lookup Table3/1, 2-D Lookup Table2/1, 2-D Lookup Table/1
  2-D Lookup Table5/1 -> Divide5/2
  Divide5/1 -> Mux1/6

== system eVTOL_PX4_2023b/Subsystem2/airframe/force moment/aero F&M in body axis/Aerodynamic Coefficients/Actuator Increments/V_right ==
  alpha : Inport
  dr : Inport  Port=2
  2-D Lookup Table : Lookup_n-D  NumberOfTableDimensions=1  BreakpointsForDimension1=aDr.alpha  BreakpointsForDimension2=aDl.alpha  BreakpointsForDimension3=aDe.flap  Table=aDr.CLDr  InternalRulePriority=Speed  RndMeth=Simplest
  2-D Lookup Table1 : Lookup_n-D  NumberOfTableDimensions=1  BreakpointsForDimension1=aDr.alpha  BreakpointsForDimension2=aDe.alpha  BreakpointsForDimension3=aDe.flap  Table=aDr.CmDr  InternalRulePriority=Speed  RndMeth=Simplest
  2-D Lookup Table2 : Lookup_n-D  NumberOfTableDimensions=1  BreakpointsForDimension1=aDr.alpha  BreakpointsForDimension2=aDe.alpha  BreakpointsForDimension3=aDe.flap  Table=aDr.CDDr  InternalRulePriority=Speed  RndMeth=Simplest
  2-D Lookup Table3 : Lookup_n-D  NumberOfTableDimensions=1  BreakpointsForDimension1=aDr.alpha  BreakpointsForDimension2=aDe.alpha  BreakpointsForDimension3=aDe.flap  Table=aDr.CYDr  InternalRulePriority=Speed  RndMeth=Simplest
  2-D Lookup Table4 : Lookup_n-D  NumberOfTableDimensions=1  BreakpointsForDimension1=aDr.alpha  BreakpointsForDimension2=aDe.alpha  BreakpointsForDimension3=aDe.flap  Table=aDr.ClDr  InternalRulePriority=Speed  RndMeth=Simplest
  2-D Lookup Table5 : Lookup_n-D  NumberOfTableDimensions=1  BreakpointsForDimension1=aDr.alpha  BreakpointsForDimension2=aDe.alpha  BreakpointsForDimension3=aDe.flap  Table=aDr.CnDr  InternalRulePriority=Speed  RndMeth=Simplest
  Divide{,1..5} (6 alike) : Product  Inputs=**
  Mux1 : Mux  Inputs=6
  dr_Coeff : Outport  VectorParamsAs1DForOutWhenUnconnected=off
  wires:
  dr/1 -> Divide5/1, Divide4/1, Divide3/1, Divide2/1, Divide1/1, Divide/1
  alpha/1 -> 2-D Lookup Table5/1, 2-D Lookup Table1/1, 2-D Lookup Table4/1, 2-D Lookup Table3/1, 2-D Lookup Table2/1, 2-D Lookup Table/1
  Divide/1 -> Mux1/1
  2-D Lookup Table5/1 -> Divide5/2
  Divide5/1 -> Mux1/6
  2-D Lookup Table1/1 -> Divide4/2
  Divide4/1 -> Mux1/5
  Divide2/1 -> Mux1/3
  2-D Lookup Table4/1 -> Divide3/2
  2-D Lookup Table/1 -> Divide/2
  2-D Lookup Table3/1 -> Divide2/2
  Mux1/1 -> dr_Coeff/1
  Divide3/1 -> Mux1/4
  2-D Lookup Table2/1 -> Divide1/2
  Divide1/1 -> Mux1/2

== system eVTOL_PX4_2023b/UAV/airframe/force moment/aero F&M in body axis/Aerodynamic Coefficients/Actuator Increments/Aileron ==
  da : Inport
  Constant1 : Constant  Value=0
  Gain : Gain  Gain=aero.CYDa
  Gain1 : Gain  Gain=aero.ClDa
  Gain2 : Gain  Gain=aero.CnDa
  Mux1 : Mux  Inputs=6
  drCoeff : Outport  VectorParamsAs1DForOutWhenUnconnected=off
  wires:
  da/1 -> Gain/1, Gain2/1, Gain1/1
  Mux1/1 -> drCoeff/1
  Gain1/1 -> Mux1/4
  Gain/1 -> Mux1/3
  Constant1/1 -> Mux1/5, Mux1/2, Mux1/1
  Gain2/1 -> Mux1/6

== system eVTOL_PX4_2023b/UAV/airframe/force moment/aero F&M in body axis/Aerodynamic Coefficients/Actuator Increments/Elevator ==
  de : Inport
  Constant1 : Constant  Value=0
  Gain : Gain  Gain=aero.CLDe
  Gain1 : Gain  Gain=aero.CDDe
  Gain2 : Gain  Gain=aero.CmDe
  Mux1 : Mux  Inputs=6
  deCoeff : Outport  VectorParamsAs1DForOutWhenUnconnected=off
  wires:
  Gain1/1 -> Mux1/2
  Gain2/1 -> Mux1/5
  Constant1/1 -> Mux1/3, Mux1/6, Mux1/4
  Mux1/1 -> deCoeff/1
  Gain/1 -> Mux1/1
  de/1 -> Gain1/1, Gain/1, Gain2/1

== system eVTOL_PX4_2023b/UAV/airframe/force moment/aero F&M in body axis/Aerodynamic Coefficients/Actuator Increments/Ruder ==
  dr : Inport
  Constant1 : Constant  Value=0
  Gain : Gain  Gain=aero.CYDr
  Gain1 : Gain  Gain=aero.ClDr
  Gain2 : Gain  Gain=aero.CnDr
  Mux1 : Mux  Inputs=6
  drCoeff : Outport  VectorParamsAs1DForOutWhenUnconnected=off
  wires:
  dr/1 -> Gain/1, Gain2/1, Gain1/1
  Mux1/1 -> drCoeff/1
  Gain1/1 -> Mux1/4
  Gain/1 -> Mux1/3
  Constant1/1 -> Mux1/5, Mux1/2, Mux1/1
  Gain2/1 -> Mux1/6

== system eVTOL_PX4_2023b/UAV/airframe/force moment/aero F&M in body axis/Aerodynamic Coefficients/Body Rate Damping/alphaDot ==
  Constant1 : Constant  Value=aero.CLAlphaDot
  Constant2 : Constant  Value=aero.CmAlphaDot
  Constant3 : Constant  Value=0
  Mux1 : Mux  Inputs=6
  delCoeff : Outport  VectorParamsAs1DForOutWhenUnconnected=off
  wires:
  Constant1/1 -> Mux1/1
  Constant2/1 -> Mux1/5
  Mux1/1 -> delCoeff/1
  Constant3/1 -> Mux1/4, Mux1/6, Mux1/3, Mux1/2

== system eVTOL_PX4_2023b/UAV/airframe/force moment/aero F&M in body axis/Aerodynamic Coefficients/Body Rate Damping/p ==
  Constant1 : Constant  Value=0
  Constant2 : Constant  Value=aero.CYp
  Constant3 : Constant  Value=aero.Clp
  Constant4 : Constant  Value=aero.Cnp
  Mux1 : Mux  Inputs=6
  delCoeff : Outport  VectorParamsAs1DForOutWhenUnconnected=off
  wires:
  Mux1/1 -> delCoeff/1
  Constant1/1 -> Mux1/1, Mux1/2, Mux1/5
  Constant4/1 -> Mux1/6
  Constant3/1 -> Mux1/4
  Constant2/1 -> Mux1/3

== system eVTOL_PX4_2023b/UAV/airframe/force moment/aero F&M in body axis/Aerodynamic Coefficients/Body Rate Damping/q ==
  Constant1 : Constant  Value=aero.CLq
  Constant2 : Constant  Value=aero.Cmq
  Constant3 : Constant  Value=0
  Mux1 : Mux  Inputs=6
  delCoeff : Outport  VectorParamsAs1DForOutWhenUnconnected=off
  wires:
  Constant3/1 -> Mux1/2, Mux1/3, Mux1/6, Mux1/4
  Mux1/1 -> delCoeff/1
  Constant2/1 -> Mux1/5
  Constant1/1 -> Mux1/1

== system eVTOL_PX4_2023b/UAV/airframe/force moment/aero F&M in body axis/Aerodynamic Coefficients/Body Rate Damping/r ==
  Constant : Constant  Value=0
  Constant1 : Constant  Value=aero.CYr
  Constant2 : Constant  Value=aero.Clr
  Constant3 : Constant  Value=aero.Cnr
  Mux1 : Mux  Inputs=6
  delCoeff : Outport  VectorParamsAs1DForOutWhenUnconnected=off
  wires:
  Constant3/1 -> Mux1/6
  Constant/1 -> Mux1/1, Mux1/2, Mux1/5
  Mux1/1 -> delCoeff/1
  Constant1/1 -> Mux1/3
  Constant2/1 -> Mux1/4

== system eVTOL_PX4_2023b/Subsystem1/Environment/Wind Models/Dryden Wind Turbulence Model (Continuous (+q -r))/Select angular rates/Interpolate rates/wind to body transformation/convert to earth coords ==
  Wind direction : Inport
  pg_l : Inport  Port=2
  qg_l : Inport  Port=3
  Demux : Demux  Outputs=2
      settings: DisplayOption=none
  Demux1 : Demux  Outputs=2
      settings: DisplayOption=none
  Mux : Mux  Inputs=2
  Mux1 : Mux  Inputs=2
  Product1 : Product  InputSameDT=on  SaturateOnIntegerOverflow=on  OutDataTypeStr=Inherit: Same as first input
  Product2 : Product  InputSameDT=on  SaturateOnIntegerOverflow=on  OutDataTypeStr=Inherit: Same as first input
  Selector : Selector  InputPortWidth=4  IndexOptions=Index vector (dialog)  Indices=[1 4]  OutputSizes=1
  Selector1 : Selector  InputPortWidth=4  IndexOptions=Index vector (dialog)  Indices=[2 3]  OutputSizes=1
  Sum : Sum  Inputs=|+-  SaturateOnIntegerOverflow=on
  Sum1 : Sum  Inputs=|++  SaturateOnIntegerOverflow=on
  Trigonometric Function : Trigonometry  Operator=sincos
  pg : Outport  VectorParamsAs1DForOutWhenUnconnected=off
  qg : Outport  Port=2  VectorParamsAs1DForOutWhenUnconnected=off
  wires:
  Trigonometric Function/1 -> Product1/1
  Trigonometric Function/2 -> Product2/2
  Selector1/1 -> Demux1/1
  Selector/1 -> Demux/1
  Mux1/1 -> Selector1/1, Selector/1
  Product1/1 -> Mux1/2
  Product2/1 -> Mux1/1
  Demux1/2 -> Sum1/2
  Demux1/1 -> Sum1/1
  Demux/2 -> Sum/2
  Demux/1 -> Sum/1
  Sum1/1 -> qg/1
  Sum/1 -> pg/1
  Mux/1 -> Product2/1, Product1/2
  qg_l/1 -> Mux/2
  pg_l/1 -> Mux/1
  Wind direction/1 -> Trigonometric Function/1
